simulink model "Modelo_Longitudinal"  (R2023a)
settings: Solver=FixedStepAuto  StartTime=0.0  StopTime=40  FixedStep=10^-3  RelTol=1e-3
undefined symbols (not defined in the file or in its folder): K, sigbuilder_block
libraries: simulink x3, simulink_extras x1
settings Model: Creator=aluno  LastModifiedBy=wenis
settings SolverCC: AlgebraicLoopSolver=TrustRegion
settings DebuggingCC: UnconnectedInputMsg=warning  UnconnectedOutputMsg=warning  UnconnectedLineMsg=warning
settings ModelReferenceCC: EnableRefExpFcnMdlSchedulingChecks=on
settings RTWCC: DLArmComputeVersion=19.05

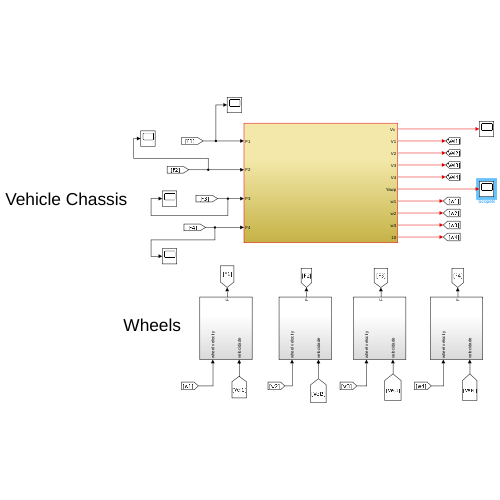
[thumbnail: Simulink's stored preview of the top-level diagram]
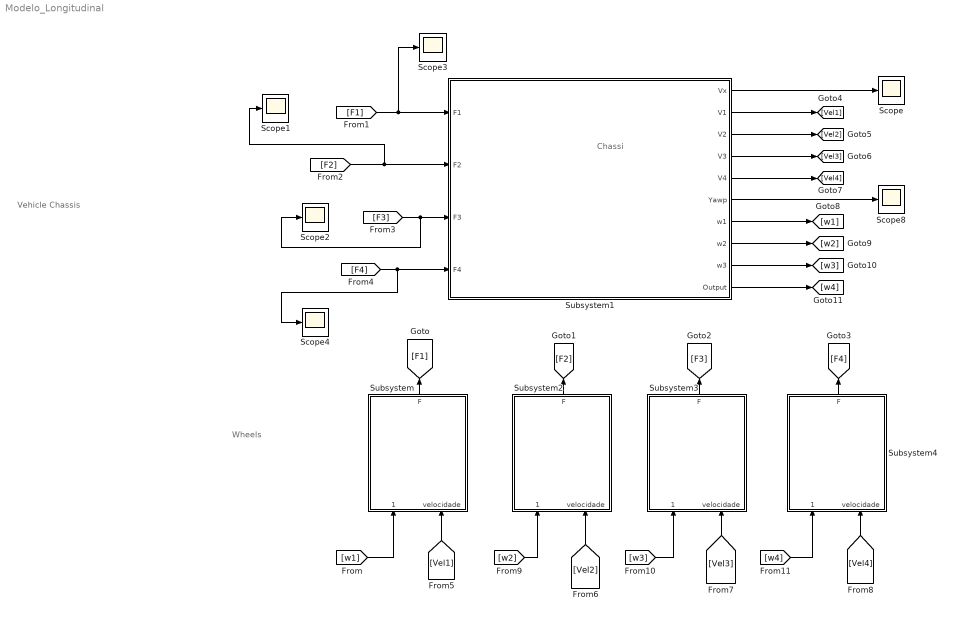
== system Modelo_Longitudinal ==
  note: Vehicle Chassis
  note: Wheels
  note: Chassi
  Scope{,1..4,8} (6 alike) : Scope
  Subsystem : Subsystem
  Subsystem1 : Subsystem
  Subsystem2 : Subsystem
  Subsystem3 : Subsystem
  Subsystem4 : Subsystem
  wires:
  [F3] -> Subsystem1/3(F3), Scope2/1
  Subsystem4/1(F) -> [F4]
  [Vel2] -> Subsystem2/2(velocidade)
  [w1] -> Subsystem/1(wheel velocity)
  Subsystem3/1(F) -> [F3]
  [F4] -> Subsystem1/4(F4), Scope4/1
  [Vel1] -> Subsystem/2(velocidade)
  [F2] -> Subsystem1/2(F2), Scope1/1
  Subsystem/1(F) -> [F1]
  Subsystem2/1(F) -> [F2]
  [F1] -> Subsystem1/1(F1), Scope3/1
  [Vel3] -> Subsystem3/2(velocidade)
  Subsystem1/6(Yawp) -> Scope8/1
  [Vel4] -> Subsystem4/2(velocidade)
  [w2] -> Subsystem2/1(wheel velocity)
  [w3] -> Subsystem3/1(wheel velocity)
  [w4] -> Subsystem4/1(wheel velocity)
  Subsystem1/1("Vx ") -> Scope/1
  Subsystem1/2(V1) -> [Vel1]
  Subsystem1/3(V2) -> [Vel2]
  Subsystem1/4(V3) -> [Vel3]
  Subsystem1/5(V4) -> [Vel4]
  Subsystem1/7(w1) -> [w1]
  Subsystem1/8(w2) -> [w2]
  Subsystem1/9(w3) -> [w3]
  Subsystem1/10(Output) -> [w4]

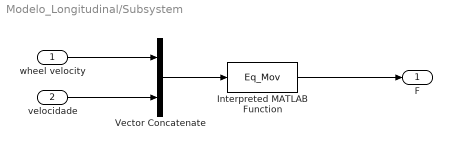
== system Modelo_Longitudinal/Subsystem ==
  wheel velocity : Inport
  velocidade : Inport  Port=2
  Interpreted MATLAB Function : MATLABFcn  MATLABFcn=Eq_Mov  OutputDimensions=2
  Vector Concatenate : Concatenate
  F : Outport
  wires:
  Vector Concatenate/1 -> Interpreted MATLAB Function/1
  velocidade/1 -> Vector Concatenate/2
  wheel velocity/1 -> Vector Concatenate/1
  Interpreted MATLAB Function/1 -> F/1

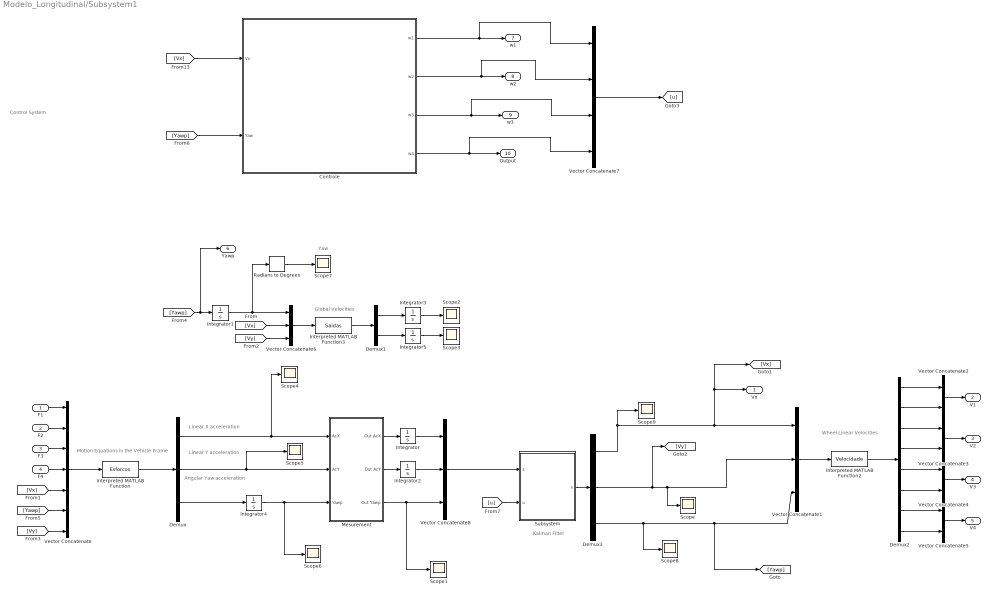
== system Modelo_Longitudinal/Subsystem1 ==
  note: Kalman Filter
  note: Yaw
  note: Wheel Linear Velocities
  note: Angular Yaw acceleration
  note: Linear X acceleration
  note: Motion Equations in the Vehicle Frame
  note: Global Velocities
  note: Linear Y acceleration
  note: Control System
  F1 : Inport
  F2 : Inport  Port=2
  F3 : Inport  Port=3
  F4 : Inport  Port=4
  Controle : Subsystem
  Demux : Demux  Outputs=3
  Demux1 : Demux  Outputs=2
  Demux2 : Demux  Outputs=8
  Demux3 : Demux  Outputs=3
  Integrator{,1..5} (6 alike) : Integrator
  Interpreted MATLAB Function : MATLABFcn  MATLABFcn=Esforcos  OutputDimensions=3
  Interpreted MATLAB Function2 : MATLABFcn  MATLABFcn=Velocidade  OutputDimensions=8
  Interpreted MATLAB Function3 : MATLABFcn  MATLABFcn=Saidas  OutputDimensions=2
  Mesurement : Subsystem
  Radians to Degrees : simulink_extras/Transformations/Radians to Degrees
  Scope{,1..9} (10 alike) : Scope
  Subsystem : Subsystem
  Vector Concatenate : Concatenate  NumInputs=7
  Vector Concatenate1 : Concatenate  NumInputs=3
  Vector Concatenate{2..5} (4 alike) : Concatenate
  Vector Concatenate6 : Concatenate  NumInputs=3
  Vector Concatenate7 : Concatenate  NumInputs=4
  Vector Concatenate8 : Concatenate  NumInputs=3
  "Vx " : Outport
  V1 : Outport  Port=2
  V2 : Outport  Port=3
  V3 : Outport  Port=4
  V4 : Outport  Port=5
  Yawp : Outport  Port=6
  w1 : Outport  Port=7
  w2 : Outport  Port=8
  w3 : Outport  Port=9
  Output : Outport  Port=10
  wires:
  Vector Concatenate/1 -> Interpreted MATLAB Function/1
  Interpreted MATLAB Function/1 -> Demux/1
  Vector Concatenate1/1 -> Interpreted MATLAB Function2/1
  Interpreted MATLAB Function2/1 -> Demux2/1
  Demux2/1 -> Vector Concatenate2/1
  Demux2/2 -> Vector Concatenate2/2
  Vector Concatenate2/1 -> V1/1
  Demux2/4 -> Vector Concatenate3/2
  Demux2/3 -> Vector Concatenate3/1
  Vector Concatenate3/1 -> V2/1
  Integrator1/1 -> Radians to Degrees/1, Vector Concatenate6/1
  Vector Concatenate6/1 -> Interpreted MATLAB Function3/1
  Interpreted MATLAB Function3/1 -> Demux1/1
  Demux1/1 -> Integrator3/1
  Demux1/2 -> Integrator5/1
  Integrator3/1 -> Scope2/1
  Integrator5/1 -> Scope3/1
  F1/1 -> Vector Concatenate/1
  F2/1 -> Vector Concatenate/2
  F3/1 -> Vector Concatenate/3
  F4/1 -> Vector Concatenate/4
  Demux/3 -> Integrator4/1
  Demux/1 -> Scope4/1, Mesurement/1(AcX)
  Demux/2 -> Scope5/1, Mesurement/2(AcY)
  Demux2/6 -> Vector Concatenate4/2
  Vector Concatenate4/1 -> V3/1
  Demux2/5 -> Vector Concatenate4/1
  Demux2/8 -> Vector Concatenate5/2
  Vector Concatenate5/1 -> V4/1
  Demux2/7 -> Vector Concatenate5/1
  [Vx] -> Vector Concatenate6/2
  [Vx] -> Vector Concatenate/5
  [Vy] -> Vector Concatenate6/3
  [Vy] -> Vector Concatenate/7
  [Yawp] -> Yawp/1, Integrator1/1
  [Yawp] -> Vector Concatenate/6
  Integrator4/1 -> Scope6/1, Mesurement/3(Yawp)
  Mesurement/1("Out AcX ") -> Integrator/1
  Mesurement/2(Out AcY) -> Integrator2/1
  Mesurement/3(Out Yawp) -> Vector Concatenate8/3, Scope1/1
  Radians to Degrees/1 -> Scope7/1
  Controle/1(w1) -> Vector Concatenate7/1, w1/1
  Controle/2(w2) -> Vector Concatenate7/2, w2/1
  [Vx] -> Controle/1(Vx)
  Controle/3(w3) -> Vector Concatenate7/3, w3/1
  Controle/4(w4) -> Vector Concatenate7/4, Output/1
  [Yawp] -> Controle/2(Yaw)
  Vector Concatenate7/1 -> [u]
  Integrator2/1 -> Vector Concatenate8/2
  Integrator/1 -> Vector Concatenate8/1
  Vector Concatenate8/1 -> Subsystem/1(z)
  [u] -> Subsystem/2(u)
  Subsystem/1(x) -> Demux3/1
  Demux3/1 -> [Vx], "Vx "/1, Vector Concatenate1/1, Scope9/1
  Demux3/3 -> Scope8/1, [Yawp], Vector Concatenate1/3
  Demux3/2 -> Scope/1, Vector Concatenate1/2, [Vy]

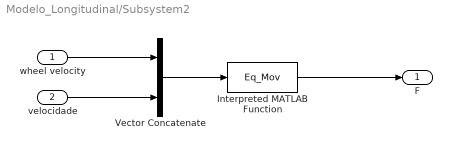
== system Modelo_Longitudinal/Subsystem2 ==
  wheel velocity : Inport
  velocidade : Inport  Port=2
  Interpreted MATLAB Function : MATLABFcn  MATLABFcn=Eq_Mov  OutputDimensions=2
  Vector Concatenate : Concatenate
  F : Outport
  wires:
  Vector Concatenate/1 -> Interpreted MATLAB Function/1
  velocidade/1 -> Vector Concatenate/2
  wheel velocity/1 -> Vector Concatenate/1
  Interpreted MATLAB Function/1 -> F/1

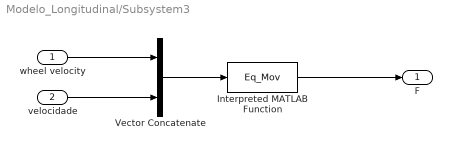
== system Modelo_Longitudinal/Subsystem3 ==
  wheel velocity : Inport
  velocidade : Inport  Port=2
  Interpreted MATLAB Function : MATLABFcn  MATLABFcn=Eq_Mov  OutputDimensions=2
  Vector Concatenate : Concatenate
  F : Outport
  wires:
  Vector Concatenate/1 -> Interpreted MATLAB Function/1
  velocidade/1 -> Vector Concatenate/2
  wheel velocity/1 -> Vector Concatenate/1
  Interpreted MATLAB Function/1 -> F/1

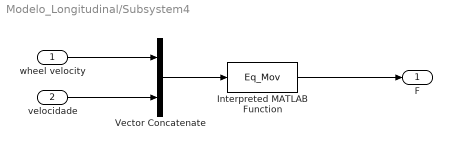
== system Modelo_Longitudinal/Subsystem4 ==
  wheel velocity : Inport
  velocidade : Inport  Port=2
  Interpreted MATLAB Function : MATLABFcn  MATLABFcn=Eq_Mov  OutputDimensions=2
  Vector Concatenate : Concatenate
  F : Outport
  wires:
  Vector Concatenate/1 -> Interpreted MATLAB Function/1
  velocidade/1 -> Vector Concatenate/2
  wheel velocity/1 -> Vector Concatenate/1
  Interpreted MATLAB Function/1 -> F/1

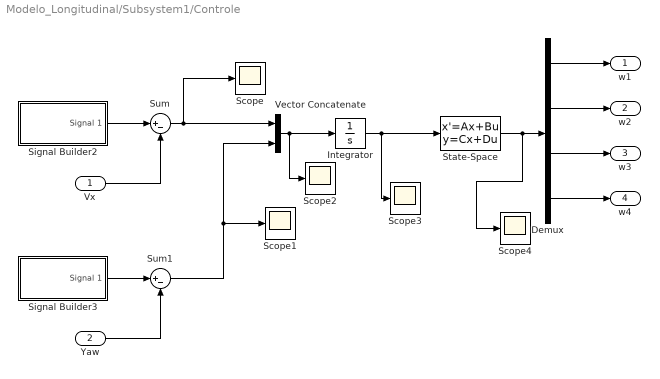
== system Modelo_Longitudinal/Subsystem1/Controle ==
  Vx : Inport
  Yaw : Inport  Port=2
  Demux : Demux
  Integrator : Integrator  InitialCondition=[0 0]
  Scope{,1..4} (5 alike) : Scope
  Signal Builder2 : Subsystem  Tag=STV Subsys  LoadFcn=sigbuilder_block('load');  StartFcn=sigbuilder_block('start');  StopFcn=sigbuilder_block('stop');  ClipboardFcn=sigbuilder_block('clipboard');  mask(Sigbuilder block){tuvar=[0:10]}
      mask help: Simulink:masks:SigbuilderBlock_MD
      mask init:
      | if ~strcmp(get_param(bdroot(gcbh),'SimulationStatus'),'stopped') tuvar = sigbuilder_block('maskInit'); end
      settings: CopyFcn=sigbuilder_block('copy');  DeleteFcn=sigbuilder_block('delete');  ModelCloseFcn=sigbuilder_block('modelClose');  PreSaveFcn=sigbuilder_block('preSave');  PauseFcn=sigbuilder_block('pause');  ContinueFcn=sigbuilder_block('continue');  NameChangeFcn=sigbuilder_block('namechange');  OpenFcn=sigbuilder_block('open',[437.25 153 550.5 359.25 ]);  CloseFcn=sigbuilder_block('close');
      mask Display: plot(0, 0, 100, 100,[2, 2, 32, 32, 2], [68, 8, 8, 68, 68],[32, 2], [38, 38], [32, 19, 2],[53, 60, 44], [32, 17, 17, 2],[16, 16, 31, 31]);txt = getActiveGroup(gcbh);text(2, 100, txt,'verticalAlignment', 'top');
  Signal Builder3 : Subsystem  Tag=STV Subsys  LoadFcn=sigbuilder_block('load');  StartFcn=sigbuilder_block('start');  StopFcn=sigbuilder_block('stop');  ClipboardFcn=sigbuilder_block('clipboard');  mask(Sigbuilder block){tuvar=[0:10]}
      mask help: Simulink:masks:SigbuilderBlock_MD
      mask init:
      | if ~strcmp(get_param(bdroot(gcbh),'SimulationStatus'),'stopped') tuvar = sigbuilder_block('maskInit'); end
      settings: CopyFcn=sigbuilder_block('copy');  DeleteFcn=sigbuilder_block('delete');  ModelCloseFcn=sigbuilder_block('modelClose');  PreSaveFcn=sigbuilder_block('preSave');  PauseFcn=sigbuilder_block('pause');  ContinueFcn=sigbuilder_block('continue');  NameChangeFcn=sigbuilder_block('namechange');  OpenFcn=sigbuilder_block('open',[326.25 94.5 558 354 ]);  CloseFcn=sigbuilder_block('close');
      mask Display: plot(0, 0, 100, 100,[2, 2, 32, 32, 2], [68, 8, 8, 68, 68],[32, 2], [38, 38], [32, 19, 2],[53, 60, 44], [32, 17, 17, 2],[16, 16, 31, 31]);txt = getActiveGroup(gcbh);text(2, 100, txt,'verticalAlignment', 'top');
  State-Space : StateSpace  A=K.A  B=K.B  C=K.C  D=K.D  InitialCondition=[0 0 0]
  Sum : Sum  Inputs=|+-
  Sum1 : Sum  Inputs=|+-
  Vector Concatenate : Concatenate
  w1 : Outport
  w2 : Outport  Port=2
  w3 : Outport  Port=3
  w4 : Outport  Port=4
  wires:
  Vx/1 -> Sum/2
  Yaw/1 -> Sum1/2
  Sum/1 -> Scope/1, Vector Concatenate/1
  Sum1/1 -> Vector Concatenate/2, Scope1/1
  Vector Concatenate/1 -> Scope2/1, Integrator/1
  Integrator/1 -> Scope3/1, State-Space/1
  State-Space/1 -> Scope4/1, Demux/1
  Demux/1 -> w1/1
  Demux/2 -> w2/1
  Demux/3 -> w3/1
  Demux/4 -> w4/1
  Signal Builder2/1(Signal 1) -> Sum/1
  Signal Builder3/1(Signal 1) -> Sum1/1

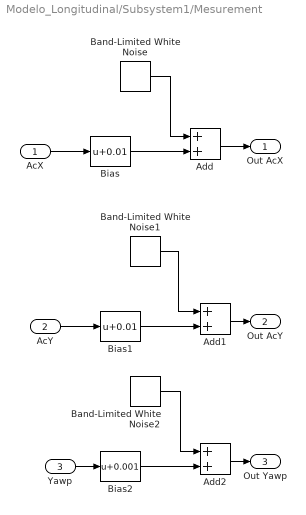
== system Modelo_Longitudinal/Subsystem1/Mesurement ==
  AcX : Inport
  AcY : Inport  Port=2
  Yawp : Inport  Port=3
  Add : Sum
  Add1 : Sum
  Add2 : Sum
  Band-Limited White Noise : simulink/Sources/Band-Limited White Noise  Cov=[0.1]  Ts=0.05  seed=[23341]
  Band-Limited White Noise1 : simulink/Sources/Band-Limited White Noise  Cov=[0.1]  Ts=0.05  seed=[23341]
  Band-Limited White Noise2 : simulink/Sources/Band-Limited White Noise  Cov=[0.001*0.001]  Ts=0.05  seed=[23341]
  Bias : Bias  Bias=0.01  SaturateOnIntegerOverflow=off
  Bias1 : Bias  Bias=0.01  SaturateOnIntegerOverflow=off
  Bias2 : Bias  Bias=0.001  SaturateOnIntegerOverflow=off
  "Out AcX " : Outport
  Out AcY : Outport  Port=2
  Out Yawp : Outport  Port=3
  wires:
  AcX/1 -> Bias/1
  Bias/1 -> Add/2
  Band-Limited White Noise/1 -> Add/1
  Add/1 -> "Out AcX "/1
  Bias1/1 -> Add1/2
  AcY/1 -> Bias1/1
  Band-Limited White Noise1/1 -> Add1/1
  Bias2/1 -> Add2/2
  Band-Limited White Noise2/1 -> Add2/1
  Yawp/1 -> Bias2/1
  Add1/1 -> Out AcY/1
  Add2/1 -> Out Yawp/1

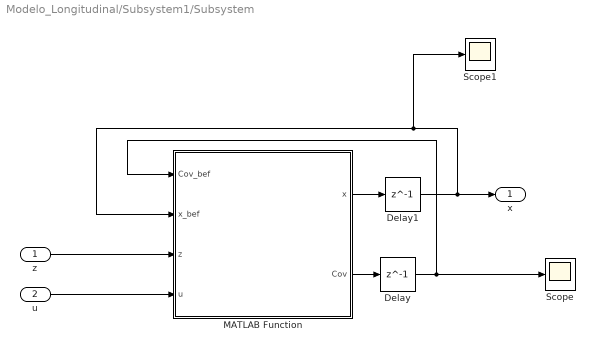
== system Modelo_Longitudinal/Subsystem1/Subsystem ==
  z : Inport
  u : Inport  Port=2
  Delay : Delay  DelayLength=1  InitialCondition=zeros(3,3)
  Delay1 : Delay  DelayLength=1  InitialCondition=[0;0;0]
  MATLAB Function : MATLAB Function  TreatAsAtomicUnit=on
  Scope : Scope
  Scope1 : Scope
  x : Outport
  wires:
  MATLAB Function/1(x) -> Delay1/1
  MATLAB Function/2(Cov) -> Delay/1
  u/1 -> MATLAB Function/4(u)
  z/1 -> MATLAB Function/3(z)
  Delay/1 -> Scope/1, MATLAB Function/1(Cov_bef)
  Delay1/1 -> x/1, Scope1/1, MATLAB Function/2(x_bef)

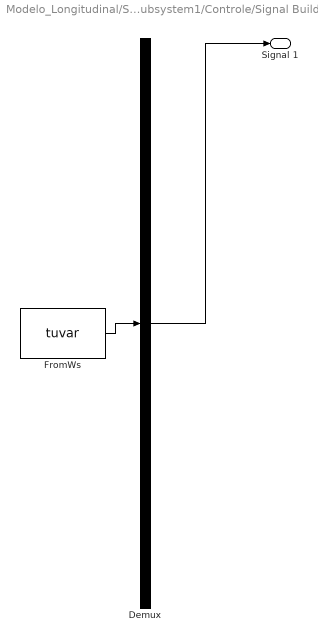
== system Modelo_Longitudinal/Subsystem1/Controle/Signal Builder2 ==
  Demux : Demux  Tag=STV Demux  Outputs=1
      settings: DisplayOption=none
  FromWs : FromWorkspace  Tag=STV FromWs  VariableName=tuvar
      SigBuilderData=|
      | common.afterFinalStr = 'Extrapolate'
      | common.sampleTime = 0
      | dataSet.timeRange = [0 10]
      | dataSet.name = 'Group 1'
      | sbobj.Groups.Name = 'Group 1'
      | sbobj.Groups.Signals.Name = 'Signal 1'
      | sbobj.Groups.Signals.XData = [0 5 5 10]
      | sbobj.Groups.Signals.YData = [0 0 0.5 0.5]
  Signal 1 : Outport  Tag=STV Outport
  wires:
  Demux/1 -> Signal 1/1
  FromWs/1 -> Demux/1

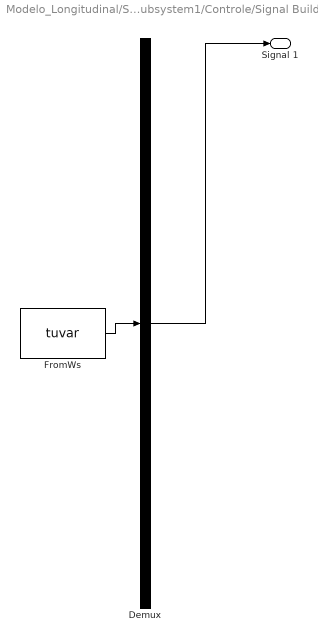
== system Modelo_Longitudinal/Subsystem1/Controle/Signal Builder3 ==
  Demux : Demux  Tag=STV Demux  Outputs=1
      settings: DisplayOption=none
  FromWs : FromWorkspace  Tag=STV FromWs  VariableName=tuvar
      SigBuilderData=|
      | common.afterFinalStr = 'Extrapolate'
      | common.sampleTime = 0
      | dataSet.timeRange = [0 10]
      | dataSet.name = 'Group 1'
      | sbobj.Groups.Name = 'Group 1'
      | sbobj.Groups.Signals.Name = 'Signal 1'
      | sbobj.Groups.Signals.XData = [0 7.02 7.02 10]
      | sbobj.Groups.Signals.YData = [0 0 0.25 0.25]
  Signal 1 : Outport  Tag=STV Outport
  wires:
  Demux/1 -> Signal 1/1
  FromWs/1 -> Demux/1

== matlab function Modelo_Longitudinal/Subsystem1/Subsystem/MATLAB Function ==
  data: Cov_bef input; x_bef input; z input; u input; x output; Cov output
function [x, Cov] = fcn(Cov_bef, x_bef,z, u)

 g=9.81;
 uc=0.7;
 vlimite=0.1;
 r=0.06;
 l=0.38/2;
 w=0.203/2;
 Iz=6.125;
 m=5.0;

Ap=[-g*uc/vlimite 0 0;
    0 g*uc/vlimite 0;
    0 0 -g*m*uc*(l^2+w^2)/(Iz*vlimite)];

   
Bp=[r*g*uc/(4*vlimite) r*g*uc/(4*vlimite) r*g*uc/(4*vlimite) r*g*uc/(4*vlimite);
    0 0 0 0;
   g*m*uc*r*w/(4*Iz*vlimite) -g*m*uc*r*w/(4*Iz*vlimite) -g*m*uc*r*w/(4*Iz*vlimite) g*m*uc*r*w/(4*Iz*vlimite)];

Cp= eye(3);

Q_k = 0.2*eye(3);
R_k = 20*eye(3);

x_belief = Ap*x_bef + Bp*u;

Cov_belief = Ap*Cov_bef*Ap' + Q_k;

%correction step
y_residue = z - Cp*x_belief;

Sk = Cp*Cov_belief*Cp' + R_k;

%Kalman gain
Kalman_Gain = Cov_belief*Cp'*(Sk)^-1;

%stimate state
x = x_belief + Kalman_Gain*y_residue;
Cov = (eye(3) - Kalman_Gain*Cp)*Cov_belief;
